simulink model "abs_CotrollModel"  (R2020a)
settings: Solver=VariableStepAuto  StartTime=0.0  StopTime=20  RelTol=1e-3
model workspace (MAT data in the model file):
  I = 6
  R = 1.25
  g = 9.8
  m = 75
  v0 = 88
undefined symbols (not defined in the file): sigbuilder_block
settings Model: EnablePacing=on  OrderedModelArguments=off  Creator=INDRAJIT MARATHE  LastModifiedBy=INDRAJIT MARATHE

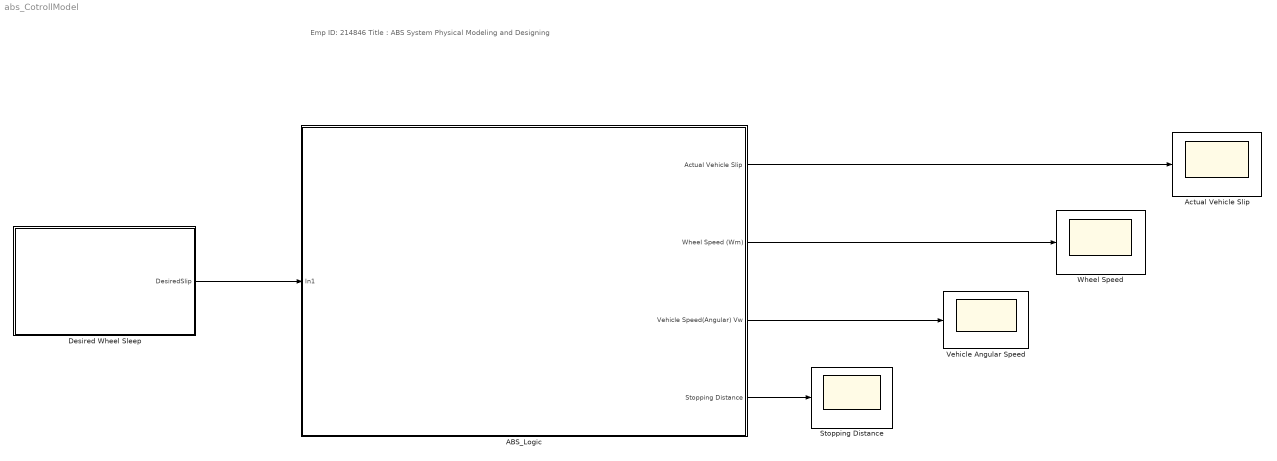
== system abs_CotrollModel ==
  note: Emp ID: 214846
      |
      | Title : ABS System Physical Modeling and Designing
  ABS_Logic : Subsystem
      mask Display: image('$imagefile'); % Use "Edit Image" on toolstrip to change.
  Actual Vehicle Slip : Scope
  Desired Wheel Sleep : Subsystem  Tag=STV Subsys  LoadFcn=sigbuilder_block('load');  StartFcn=sigbuilder_block('start');  StopFcn=sigbuilder_block('stop');  ClipboardFcn=sigbuilder_block('clipboard');  mask(Sigbuilder block){tuvar=[0:10]}
      mask help: Simulink:masks:SigbuilderBlock_MD
      mask init:
      | if ~strcmp(get_param(bdroot(gcbh),'SimulationStatus'),'stopped') tuvar = sigbuilder_block('maskInit'); end
      settings: CopyFcn=sigbuilder_block('copy');  DeleteFcn=sigbuilder_block('delete');  ModelCloseFcn=sigbuilder_block('modelClose');  PreSaveFcn=sigbuilder_block('preSave');  PauseFcn=sigbuilder_block('pause');  ContinueFcn=sigbuilder_block('continue');  NameChangeFcn=sigbuilder_block('namechange');  OpenFcn=sigbuilder_block('open',[437.6 199.2 550.4 400 ]);  CloseFcn=sigbuilder_block('close');
      mask Display: plot(0, 0, 100, 100,[2, 2, 32, 32, 2], [68, 8, 8, 68, 68],[32, 2], [38, 38], [32, 19, 2],[53, 60, 44], [32, 17, 17, 2],[16, 16, 31, 31]);txt = getActiveGroup(gcbh);text(2, 100, txt,'verticalAlignment', 'top');
  Stopping Distance : Scope
  Vehicle Angular Speed : Scope
  Wheel Speed : Scope
  wires:
  Desired Wheel Sleep/1(DesiredSlip) -> ABS_Logic/1(In1)
  ABS_Logic/2(Wheel Speed (Wm)) -> Wheel Speed/1
  ABS_Logic/3(Vehicle Speed(Angular) Vw) -> Vehicle Angular Speed/1
  ABS_Logic/4(Stopping Distance) -> Stopping Distance/1
  ABS_Logic/1(Actual Vehicle Slip) -> Actual Vehicle Slip/1

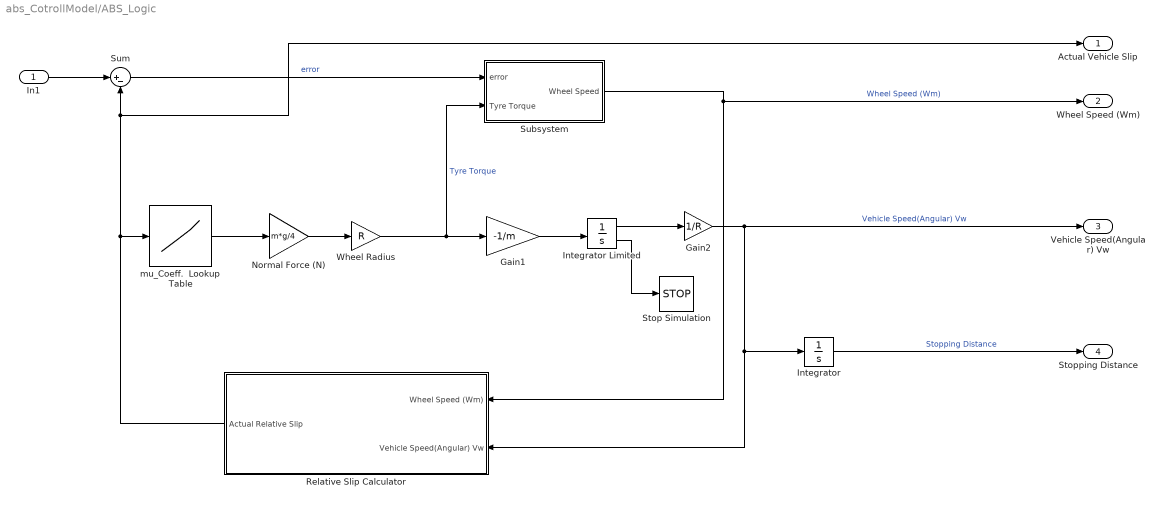
== system abs_CotrollModel/ABS_Logic ==
  In1 : Inport
  Gain1 : Gain  Gain=-1/m
  Gain2 : Gain  Gain=1/R
  Integrator : Integrator
  Integrator Limited : Integrator  InitialCondition=v0  LimitOutput=on  UpperSaturationLimit=1000  LowerSaturationLimit=0  ShowSaturationPort=on
  Normal Force (N) : Gain  Gain=m*g/4
  Relative Slip Calculator : Subsystem
  Stop Simulation : Stop
  Subsystem : Subsystem
  Sum : Sum  Inputs=|+-
  Wheel Radius : Gain  Gain=R
  mu_Coeff.  Lookup Table : Lookup_n-D  NumberOfTableDimensions=1  BreakpointsForDimension1=[0,0.05,0.1,0.15,0.2,0.25,0.3,0.35,0.4,0.45,0.5,0.55,0.6,0.65,0.7,0.75,0.8,0.85,0.9,0.95,1]  BreakpointsForDimension1FirstPoint=0  BreakpointsForDimension1Spacing=0.05  Table=[0,0.4,0.8,0.97,1,0.98,0.96,0.94,0.92,0.9,0.88,0.85,0.83,0.81,0.79,0.77,0.75,0.73,0.72,0.71,0.7]  InternalRulePriority=Speed  RndMeth=Simplest  InputSameDT=on
  Actual Vehicle Slip : Outport
  Wheel Speed (Wm) : Outport  Port=2
  Vehicle Speed(Angular) Vw : Outport  Port=3
  Stopping Distance : Outport  Port=4
  wires:
  Wheel Radius/1 -> Subsystem/2(Tyre Torque), Gain1/1  "Tyre Torque"
  Integrator Limited/2 -> Stop Simulation/1
  Gain2/1 -> Vehicle Speed(Angular) Vw/1, Relative Slip Calculator/2(Vehicle Speed(Angular) Vw), Integrator/1  "Vehicle Speed(Angular) Vw"
  Relative Slip Calculator/1(Actual Relative Slip) -> mu_Coeff.  Lookup Table/1, Sum/2, Actual Vehicle Slip/1
  Integrator Limited/1 -> Gain2/1
  mu_Coeff.  Lookup Table/1 -> Normal Force (N)/1
  Normal Force (N)/1 -> Wheel Radius/1
  Gain1/1 -> Integrator Limited/1
  Subsystem/1(Wheel Speed) -> Wheel Speed (Wm)/1, Relative Slip Calculator/1(Wheel Speed (Wm))  "Wheel Speed (Wm)"
  Sum/1 -> Subsystem/1(error)  "error"
  Integrator/1 -> Stopping Distance/1  "Stopping Distance"
  In1/1 -> Sum/1

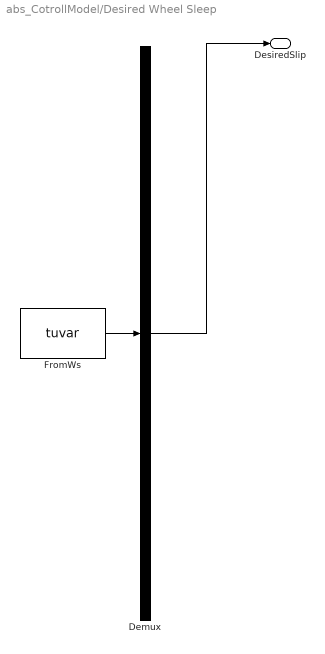
== system abs_CotrollModel/Desired Wheel Sleep ==
  Demux : Demux  Tag=STV Demux  Outputs=1
      settings: DisplayOption=none
  FromWs : FromWorkspace  Tag=STV FromWs  VariableName=tuvar
      SigBuilderData=|
      | common.afterFinalStr = 'Extrapolate'
      | common.sampleTime = 0
      | dataSet.timeRange = [0 10]
      | dataSet.name = 'Group 1'
      | sbobj.Groups.Name = 'Group 1'
      | sbobj.Groups.Signals.Name = 'DesiredSlip'
      | sbobj.Groups.Signals.XData = [0 10]
      | sbobj.Groups.Signals.YData = [0.2 0.2]
  DesiredSlip : Outport  Tag=STV Outport
  wires:
  FromWs/1 -> Demux/1
  Demux/1 -> DesiredSlip/1

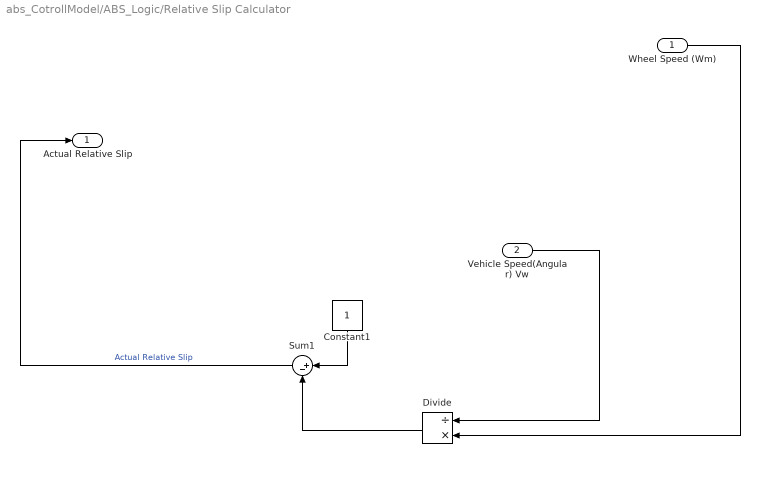
== system abs_CotrollModel/ABS_Logic/Relative Slip Calculator ==
  Wheel Speed (Wm) : Inport
  Vehicle Speed(Angular) Vw : Inport  Port=2
  Constant1 : Constant
  Divide : Product  Inputs=/*
  Sum1 : Sum  Inputs=|+-
  Actual Relative Slip : Outport
  wires:
  Wheel Speed (Wm)/1 -> Divide/2
  Divide/1 -> Sum1/2
  Vehicle Speed(Angular) Vw/1 -> Divide/1
  Sum1/1 -> Actual Relative Slip/1  "Actual Relative Slip"
  Constant1/1 -> Sum1/1

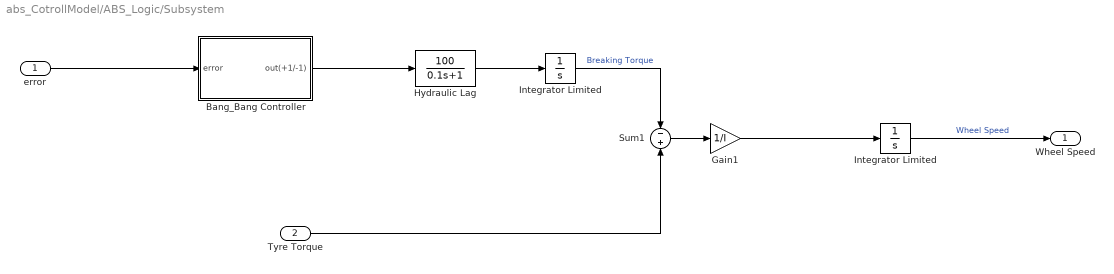
== system abs_CotrollModel/ABS_Logic/Subsystem ==
  error : Inport
  Tyre Torque : Inport  Port=2
  " Integrator Limited" : Integrator  LimitOutput=on  UpperSaturationLimit=1000  LowerSaturationLimit=0
  Bang_Bang Controller : Subsystem
  Gain1 : Gain  Gain=1/I
  "Hydraulic Lag " : TransferFcn  Numerator=[100]  Denominator=[0.1 1]
  Integrator Limited : Integrator  InitialCondition=v0/R  LimitOutput=on  UpperSaturationLimit=1000  LowerSaturationLimit=0
  Sum1 : Sum  Inputs=-+
  Wheel Speed : Outport
  wires:
  Bang_Bang Controller/1(out(+1/-1)) -> "Hydraulic Lag "/1
  error/1 -> Bang_Bang Controller/1(error)
  Sum1/1 -> Gain1/1
  " Integrator Limited"/1 -> Sum1/1  "Breaking Torque"
  Tyre Torque/1 -> Sum1/2
  "Hydraulic Lag "/1 -> " Integrator Limited"/1
  Gain1/1 -> Integrator Limited/1
  Integrator Limited/1 -> Wheel Speed/1  "Wheel Speed"

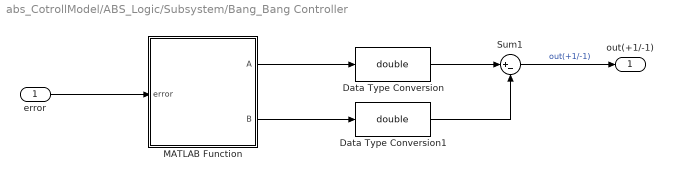
== system abs_CotrollModel/ABS_Logic/Subsystem/Bang_Bang Controller ==
  error : Inport
  Data Type Conversion : DataTypeConversion  OutDataTypeStr=double  RndMeth=Zero
  Data Type Conversion1 : DataTypeConversion  OutDataTypeStr=double  RndMeth=Zero
  MATLAB Function : MATLAB Function  TreatAsAtomicUnit=on
  Sum1 : Sum  Inputs=|+-
  out(+1/-1) : Outport
  wires:
  Sum1/1 -> out(+1/-1)/1  "out(+1/-1)"
  Data Type Conversion1/1 -> Sum1/2
  MATLAB Function/2(B) -> Data Type Conversion1/1
  error/1 -> MATLAB Function/1(error)
  Data Type Conversion/1 -> Sum1/1
  MATLAB Function/1(A) -> Data Type Conversion/1

== matlab function abs_CotrollModel/ABS_Logic/Subsystem/Bang_Bang Controller/MATLAB Function ==
  data: error input; A output; B output
function [A,B]= fcn(error)
 if error>0
     A=1;
     B=0;
 else
     A=0;
     B=1;
 end;
